simulink library "library_BCM"  (Simulink 8.2)
settings: Solver=ode45  StartTime=0.0  StopTime=10.0  RelTol=1e-3
undefined symbols (not defined in the file or in its folder): MPU_FOUR_CST, MPU_ONE_CST, MPU_THREE_CST, MPU_TWO_CST, MPU_ZERO_CST, NAMEOFTHEMODEL_SAMPLE_TIME_CST, slcm, TYP_MPU_REQUEST, TYP_MPU_REQUEST_2, TYP_MPU_STATUS, TYP_MPU_STATUS_2
libraries: Renault_Library x50, simulink x8, library_BCM x7
(part 2 of 3)

== system library_BCM/Modeling/PRESOAK_CHARGE_5CAL_7DAY ==
  IN_Prog_time : Inport
  CURENT_TIME : Inport  Port=2
  ONE_WEEK_IN_MINUTES : Inport  Port=3
  RelationalOperator : RelationalOperator  Operator=>  OutDataTypeStr=boolean  InputSameDT=on
  Subtract : Sum  Inputs=+-  OutDataTypeStr=Inherit: Inherit via back propagation  RndMeth=Zero  InputSameDT=on
  Sum : Sum  Inputs=++-  OutDataTypeStr=Inherit: Inherit via back propagation  RndMeth=Zero  InputSameDT=on
  Switch1 : Switch  Criteria=u2 ~= 0  RndMeth=Zero  InputSameDT=on
      settings: AttributesFormatString=Criteria=%<Criteria>
  Out_WUP : Outport
  wires:
  ONE_WEEK_IN_MINUTES/1 -> Sum/2
  Switch1/1 -> Out_WUP/1
  Sum/1 -> Switch1/3
  [CURENT_TIME] -> Sum/3
  [Prog_time] -> Sum/1
  [CURENT_TIME] -> Subtract/2
  [Prog_time] -> Subtract/1
  Subtract/1 -> Switch1/1
  IN_Prog_time/1 -> [Prog_time]
  CURENT_TIME/1 -> [CURENT_TIME]
  [CURENT_TIME] -> RelationalOperator/2
  RelationalOperator/1 -> Switch1/2
  [Prog_time] -> RelationalOperator/1

== system library_BCM/Modeling/RSA_Dynamic2DLookupTable_V01_00 ==
  x : Inport
  y : Inport  Port=2
  x_breakpoints : Inport  Port=3
  y_breakpoints : Inport  Port=4
  table : Inport  Port=5
  InterpolationUsingPrelookup : Interpolation_n-D  TableSource=Input port  ExtrapMethod=Clip  RndMeth=Zero
      settings: InputPortMap=u0,u1,u2,u3,p2
  Prelookup : PreLookup  BreakpointsDataSource=Input port  BreakpointsData=[1:4]  RndMeth=Zero
      settings: InputPortMap=u0,p1
  Prelookup1 : PreLookup  BreakpointsDataSource=Input port  BreakpointsData=[1:4]  RndMeth=Zero
      settings: InputPortMap=u0,p1
  Out : Outport
  wires:
  x/1 -> Prelookup/1
  InterpolationUsingPrelookup/1 -> Out/1
  table/1 -> InterpolationUsingPrelookup/5
  y/1 -> Prelookup1/1
  x_breakpoints/1 -> Prelookup/2
  y_breakpoints/1 -> Prelookup1/2
  Prelookup/2 -> InterpolationUsingPrelookup/2
  Prelookup/1 -> InterpolationUsingPrelookup/1
  Prelookup1/2 -> InterpolationUsingPrelookup/4
  Prelookup1/1 -> InterpolationUsingPrelookup/3

== system library_BCM/Modeling/TIME_OUT ==
  In : Inport  OutDataTypeStr=boolean
  dly : Inport  Port=2
  Constant1 : Constant  OutDataTypeStr=Inherit: Inherit via back propagation  SampleTime=-1
  Constant4 : Constant  Value=Ps  SampleTime=-1
  Constant9 : Constant  Value=INIVAL  SampleTime=-1
  DataTypeConversion : DataTypeConversion  OutDataTypeStr=uint32  RndMeth=Zero
  LogicalOperator1 : Logic  Operator=NOT  OutDataTypeStr=boolean
  MinMax : MinMax  Tag=AM,Std,Inputs,1;CMP,Function,Inputs;  Inputs=2  OutDataTypeStr=Inherit: Inherit via back propagation  RndMeth=Zero  SaturateOnIntegerOverflow=on  InputSameDT=on
  MinMax1 : MinMax  Tag=AM,Std,Inputs,1;CMP,Function,Inputs;  Function=max  Inputs=2  OutDataTypeStr=Inherit: Inherit via back propagation  RndMeth=Zero  SaturateOnIntegerOverflow=on  InputSameDT=on
  RSA_DetectDecrease : Renault_Library/Complex blocks/Logic & Bit Operations/RSA_DetectDecrease  Tag=[LIB]  vinit=false
      settings: AttributesFormatString=%<MaskType> : Ver : 01.02\nInitial condition: %<vinit>
  RelationalOperator1 : RelationalOperator  Tag=AM,Std,2,1;CMP,Operator;  Operator===  OutDataTypeStr=boolean  InputSameDT=on
  Sum1 : Sum  OutDataTypeStr=Inherit: Inherit via back propagation  RndMeth=Zero  SaturateOnIntegerOverflow=on  InputSameDT=on
  Sum2 : Sum  Inputs=+-  OutDataTypeStr=Inherit: Inherit via back propagation  RndMeth=Zero  SaturateOnIntegerOverflow=on  InputSameDT=on
  Sum3 : Sum  Inputs=+-  OutDataTypeStr=Inherit: Inherit via back propagation  RndMeth=Zero  SaturateOnIntegerOverflow=on  InputSameDT=on
  Switch1 : Switch  Criteria=u2 ~= 0  RndMeth=Zero  SaturateOnIntegerOverflow=on  InputSameDT=on
      settings: AttributesFormatString=Criteria=%<Criteria>
  UnitDelay : UnitDelay  InitialCondition=InitialConditions  SampleTime=-1
      settings: AttributesFormatString=IC = %<X0>
  UnitDelay1 : UnitDelay  InitialCondition=UDVAL  SampleTime=-1
      settings: AttributesFormatString=IC = %<X0>
  Out : Outport
  wires:
  Constant1/1 -> Sum3/2
  Sum3/1 -> DataTypeConversion/1
  dly/1 -> Sum3/1
  UnitDelay/1 -> Out/1
  LogicalOperator1/1 -> RSA_DetectDecrease/1
  RelationalOperator1/1 -> LogicalOperator1/1
  MinMax1/1 -> RelationalOperator1/1
  [Nsx_Zero] -> RelationalOperator1/2, MinMax1/2
  Sum2/1 -> MinMax/2
  MinMax/1 -> MinMax1/1
  In/1 -> Switch1/2
  Constant9/1 -> [Nsx_Zero], Switch1/1
  Sum1/1 -> Switch1/3
  UnitDelay1/1 -> Sum1/2
  Switch1/1 -> Sum2/2, UnitDelay1/1
  Constant4/1 -> Sum1/1
  DataTypeConversion/1 -> MinMax/1, Sum2/1
  RSA_DetectDecrease/1 -> UnitDelay/1

== system library_BCM/Modeling/Timer_Conversion ==
  TIMER_TO_ADAPT : Inport
      settings: AttributesFormatString=Type : %<OutDataTypeStr>
  Constant1 : Constant  Value=NAMEOFTHEMODEL_SAMPLE_TIME_CST  OutDataTypeStr=uint8  SampleTime=-1
  Constant2 : Constant  Value=NAMEOFTHEMODEL_SAMPLE_TIME_CST  OutDataTypeStr=Inherit: Inherit via back propagation  SampleTime=-1
  Constant3 : Constant  Value=ZERO_CST  OutDataTypeStr=Inherit: Inherit via back propagation  SampleTime=-1
  Divide : Product  Inputs=*/  SaturateOnIntegerOverflow=on  RndMeth=Zero  InputSameDT=on
      settings: AttributesFormatString=Saturation:%<SaturateOnIntegerOverflow>
  RelationalOperator1 : RelationalOperator  Operator===  OutDataTypeStr=boolean  InputSameDT=on
  Switch : Switch  Criteria=u2 ~= 0  RndMeth=Zero  InputSameDT=on
      settings: AttributesFormatString=Criteria=%<Criteria>
  TIMER_ADAPTED : Outport
      settings: AttributesFormatString=Type : %<OutDataTypeStr>\nInit :%<InitialOutput>
  wires:
  Divide/1 -> Switch/3
  [TIMER_TO_ADAPT] -> Divide/1
  [TIMER_TO_ADAPT] -> Switch/1
  TIMER_TO_ADAPT/1 -> [TIMER_TO_ADAPT]
  Switch/1 -> TIMER_ADAPTED/1
  RelationalOperator1/1 -> Switch/2
  Constant3/1 -> RelationalOperator1/2
  Constant1/1 -> RelationalOperator1/1
  Constant2/1 -> Divide/2

== system library_BCM/Validation/EEPROM ==
  EEPROM_S : Inport
  EEPROM_S_OUT : Inport  Port=2
  ECU_RESET : Inport  Port=3
  Data Store Memory : DataStoreMemory  DataStoreName=EEPROM_S  ReadBeforeWriteMsg=warning  WriteAfterWriteMsg=warning  WriteAfterReadMsg=warning
  DataStoreRead : Subsystem
      mask Display: fprintf('DataStoreRead')
  DataStoreWrite : Subsystem
      mask Display: fprintf('DataStoreWrite')
  EEPROM_S_IN : Outport
  wires:
  DataStoreRead/1(EEPROM_S_N) -> EEPROM_S_IN/1
  EEPROM_S_OUT/1 -> DataStoreWrite/2(EEPROM_S_OUT)
  EEPROM_S/1 -> DataStoreWrite/1(EEPROM_S)
  ECU_RESET/1 -> DataStoreWrite/3(ECU_RESET)

== system library_BCM/Validation/EEPROM_OLD ==
  READ : Inport
  WRITE : Inport  Port=2
  Chart : Stateflow chart  TreatAsAtomicUnit=on
  MultiportSwitch : MultiPortSwitch  Inputs=2
  S_IN : Outport
  wires:
  Chart/1(x) -> MultiportSwitch/1
  READ/1 -> MultiportSwitch/2, Chart/1(READ)
  WRITE/1 -> MultiportSwitch/3, Chart/2(WRITE)
  MultiportSwitch/1 -> S_IN/1

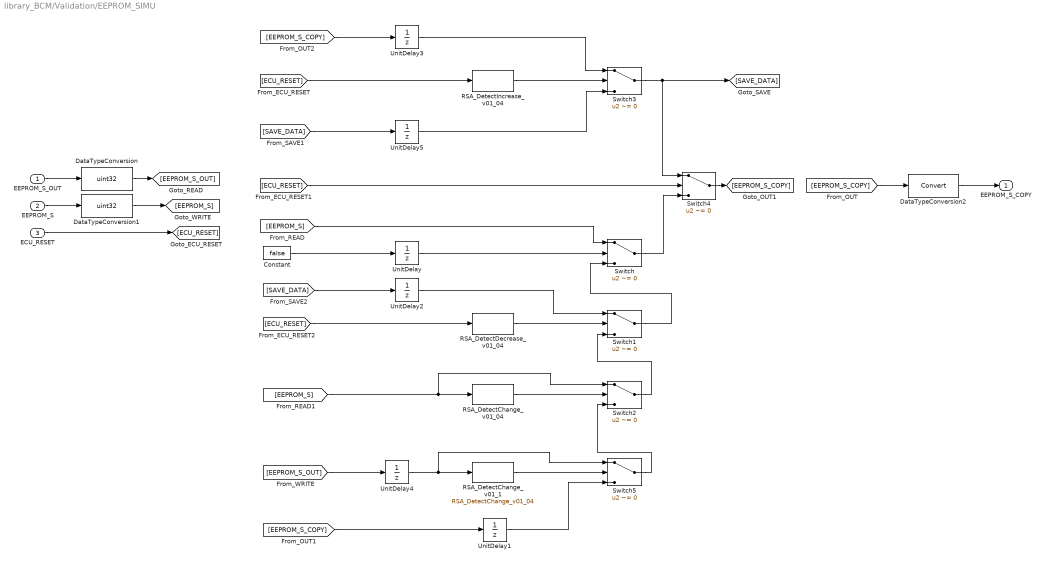
== system library_BCM/Validation/EEPROM_SIMU ==
  EEPROM_S_OUT : Inport
  EEPROM_S : Inport  Port=2
  ECU_RESET : Inport  Port=3
  Constant : Constant  Value=false  OutDataTypeStr=boolean  SampleTime=-1
  DataTypeConversion : DataTypeConversion  OutDataTypeStr=uint32  RndMeth=Zero
      settings: AttributesFormatString=Saturation:%<SaturateOnIntegerOverflow>
  DataTypeConversion1 : DataTypeConversion  OutDataTypeStr=uint32  RndMeth=Zero
      settings: AttributesFormatString=Saturation:%<SaturateOnIntegerOverflow>
  DataTypeConversion2 : DataTypeConversion  RndMeth=Zero
      settings: AttributesFormatString=Saturation:%<SaturateOnIntegerOverflow>
  RSA_DetectChange_v01_04 : Renault_Library/Complex blocks/Logic & Bit Operations/RSA_DetectChange_v01_04  Tag=[LIB]  chkini=off  vinit=0
      settings: AttributesFormatString=%<MaskType> : Ver : 01.04\nCompare the Input with Initial Value = %<chkini>\nInitial Value : = %<vinit>
  RSA_DetectChange_v01_1 : Renault_Library/Complex blocks/Logic & Bit Operations/RSA_DetectChange_v01_04  Tag=[LIB]  chkini=off  vinit=0
      settings: AttributesFormatString=%<MaskType> : Ver : 01.04\nCompare the Input with Initial Value = %<chkini>\nInitial Value : = %<vinit>
  RSA_DetectDecrease_v01_04 : Renault_Library/Complex blocks/Logic & Bit Operations/RSA_DetectDecrease_v01_04  Tag=[LIB]  chkini=on  vinit=0
      settings: AttributesFormatString=%<MaskType> : Ver : 01.04\nCompare the Input with Initial Value = %<chkini>\nInitial Value : = %<vinit>
  RSA_DetectIncrease_v01_04 : Renault_Library/Complex blocks/Logic & Bit Operations/RSA_DetectIncrease_v01_04  Tag=[LIB]  chkini=off  vinit=false
      settings: AttributesFormatString=%<MaskType> : Ver : 01.04\nCompare the Input with Initial Value = %<chkini>\nInitial Value : = %<vinit>
  Switch{,1..5} (6 alike) : Switch  Criteria=u2 ~= 0  RndMeth=Zero  InputSameDT=on
      settings: AttributesFormatString=Criteria=%<Criteria>
  UnitDelay : UnitDelay  InitialCondition=true  SampleTime=-1
      settings: AttributesFormatString=IC = %<X0>
  UnitDelay{1..5} (5 alike) : UnitDelay  SampleTime=-1
      settings: AttributesFormatString=IC = %<X0>
  EEPROM_S_COPY : Outport
  wires:
  DataTypeConversion2/1 -> EEPROM_S_COPY/1
  DataTypeConversion1/1 -> [EEPROM_S]
  DataTypeConversion/1 -> [EEPROM_S_OUT]
  [ECU_RESET] -> Switch4/2
  Switch/1 -> Switch4/3
  UnitDelay5/1 -> Switch3/3
  [SAVE_DATA] -> UnitDelay5/1
  UnitDelay3/1 -> Switch3/1
  RSA_DetectIncrease_v01_04/1 -> Switch3/2
  Switch3/1 -> [SAVE_DATA], Switch4/1
  Switch4/1 -> [EEPROM_S_COPY]
  [EEPROM_S_COPY] -> UnitDelay3/1
  [ECU_RESET] -> RSA_DetectIncrease_v01_04/1
  ECU_RESET/1 -> [ECU_RESET]
  EEPROM_S/1 -> DataTypeConversion1/1
  EEPROM_S_OUT/1 -> DataTypeConversion/1
  [EEPROM_S_COPY] -> DataTypeConversion2/1
  Constant/1 -> UnitDelay/1
  UnitDelay/1 -> Switch/2
  [EEPROM_S] -> Switch/1
  RSA_DetectChange_v01_04/1 -> Switch2/2
  [EEPROM_S] -> Switch2/1, RSA_DetectChange_v01_04/1
  [ECU_RESET] -> RSA_DetectDecrease_v01_04/1
  RSA_DetectDecrease_v01_04/1 -> Switch1/2
  [SAVE_DATA] -> UnitDelay2/1
  UnitDelay2/1 -> Switch1/1
  Switch1/1 -> Switch/3
  Switch2/1 -> Switch1/3
  [EEPROM_S_OUT] -> UnitDelay4/1
  RSA_DetectChange_v01_1/1 -> Switch5/2
  Switch5/1 -> Switch2/3
  [EEPROM_S_COPY] -> UnitDelay1/1
  UnitDelay1/1 -> Switch5/3
  UnitDelay4/1 -> Switch5/1, RSA_DetectChange_v01_1/1

== system library_BCM/Fault Manager/DTC/DETECT_DTC_IN_E2P_FOR_RESET ==
  FailureConfirmed : Inport  OutDataTypeStr=boolean
      settings: AttributesFormatString=Type : %<OutDataTypeStr>
  DTC_LIST_OUT_EXT_DATA_S : Inport  Port=2  OutDataTypeStr=uint32
      settings: AttributesFormatString=Type : %<OutDataTypeStr>
  NUMBER_DTC_RECORD_IN_E2P_CST : Inport  Port=3  OutDataTypeStr=uint32
      settings: AttributesFormatString=Type : %<OutDataTypeStr>
  DTC_LIST_OUT_IDENTITY_DTC_S : Inport  Port=4  OutDataTypeStr=uint32
      settings: AttributesFormatString=Type : %<OutDataTypeStr>
  DTC_ID : Inport  Port=5  OutDataTypeStr=uint32
      settings: AttributesFormatString=Type : %<OutDataTypeStr>
  Enable : EnablePort
      settings: AttributesFormatString=State : %<StatesWhenEnabling>
  ForIteratorSubsystem : Subsystem  TreatAsAtomicUnit=on
  TO_ADD_1_CALCUL_IN_LOOP : Subsystem
  ExtendedData_reset : Outport  OutDataTypeStr=uint32  InitialOutput=0
      settings: CopyFcn=if exist('tl_check_ports','file'), tl_check_ports(gcbh); end  NameChangeFcn=if exist('tl_check_ports','file'), tl_check_ports(gcbh); end
  wires:
  FailureConfirmed/1 -> ForIteratorSubsystem/5(FailureConfirmed)
  DTC_ID/1 -> ForIteratorSubsystem/4(DTC_ID)
  DTC_LIST_OUT_IDENTITY_DTC_S/1 -> ForIteratorSubsystem/3(DTC_LIST_OUT_IDENTITY_DTC_S)
  DTC_LIST_OUT_EXT_DATA_S/1 -> ForIteratorSubsystem/2(DTC_LIST_OUT_EXT_DATA_S)
  ForIteratorSubsystem/1(ExtendedData) -> ExtendedData_reset/1
  TO_ADD_1_CALCUL_IN_LOOP/1(NB_DTC_RECORD_IN_E2P_CST_EXT) -> [NB_DTC_RECORD_IN_E2P_CST_EXT]
  NUMBER_DTC_RECORD_IN_E2P_CST/1 -> TO_ADD_1_CALCUL_IN_LOOP/1(NUMBER_DTC_RECORD_IN_E2P_CST)
  [NB_DTC_RECORD_IN_E2P_CST_EXT] -> ForIteratorSubsystem/1(NUMBER_DTC_RECORD_IN_E2P_CST)

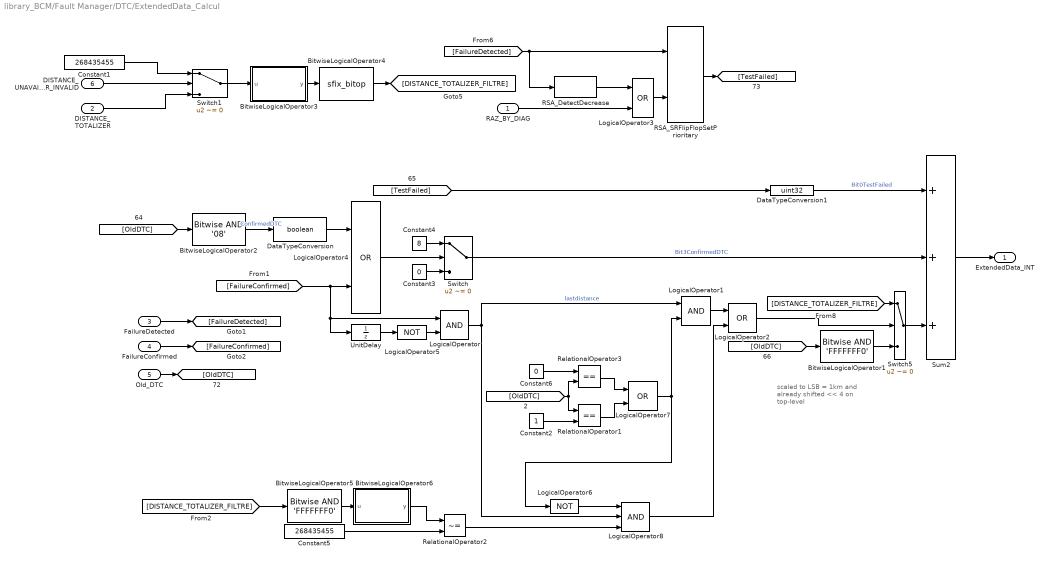
== system library_BCM/Fault Manager/DTC/ExtendedData_Calcul ==
  note: scaled to LSB = 1km
      | and already shifted << 4
      | on top-level
  RAZ_BY_DIAG : Inport  OutDataTypeStr=boolean
  DISTANCE_TOTALIZER : Inport  Port=2  OutDataTypeStr=uint32
      settings: CopyFcn=if exist('tl_check_ports','file'), tl_check_ports(gcbh); end  NameChangeFcn=if exist('tl_check_ports','file'), tl_check_ports(gcbh); end
  FailureDetected : Inport  Port=3  OutDataTypeStr=boolean
  FailureConfirmed : Inport  Port=4  OutDataTypeStr=boolean
  Old_DTC : Inport  Port=5  OutDataTypeStr=uint32
  DISTANCE_UNAVAILABLE_OR_INVALID : Inport  Port=6  OutDataTypeStr=boolean
  BitwiseLogicalOperator1 : simulink/Logic and Bit Operations/Bitwise Operator  Tag=struct('revisionNumber',2,'output',struct('type','UInt32'),'operator','AND','operand2','''FFFFFF00''','numInput',1)  logicop=AND  UseBitMask=on  BitMask='FFFFFFF0'  BitMaskRealWorld=Stored Integer
  BitwiseLogicalOperator2 : simulink/Logic and Bit Operations/Bitwise Operator  Tag=struct('revisionNumber',2,'output',struct('type','UInt8'),'operator','AND','operand2','''08''','numInput',1)  logicop=AND  UseBitMask=on  BitMask='08'  BitMaskRealWorld=Stored Integer
  BitwiseLogicalOperator3 : Subsystem  Tag=struct('revisionNumber',2,'output',struct('type','UInt32'),'operator','SHIFT_LEFT','operand2','8','numInput',1)  mask(Shift Arithmetic){nBitShiftRight=-4, nBinPtShiftRight=0}
      mask prompts: nBitShiftRight "Number of bits to shift right (use negative value to shift left):"; nBinPtShiftRight "Number of places by which binary point shifts right (use negative value to shift left):"
      mask help:
      | This block can arithmetically shift the bits and/or the binary point of a signal.
      | The effect of these actions can be interpreted as a combination of a multiplication by a power of two and a change in scaling.  The power of two multiplication term is
      |   2^( NumBinaryPointShiftsRight - NumBitShiftsRight )
      | Negative values for shifts right are actually positive shift lefts.
      | If the input is a floating point type, the power of two multiplication is carried out, but no change in scaling is applied.
      mask init:
      | netExponent = nBinPtShiftRight - nBitShiftRight;
      | netExponent(find(netExponent>127)) = 127;
      | netExponent(find(netExponent<-127)) = -127;
      | nBitShiftRight(find(nBitShiftRight>127)) = 127;
      | nBitShiftRight(find(nBitShiftRight<-127)) = -127;
      | dstr = ['Vy = Vu'];
      | if netExponent ~= 0
      |   dstr = [dstr,' * 2^',num2str(netExponent)];
      | end
      | dstr = [dstr,'\nQy = Qu'];
      | if nBitShiftRight > 0
      |   dstr = [dstr,' >> ',num2str(nBitShiftRight)];
      | elseif nBitShiftRight < 0
      |  dstr = [dstr,' << ',num2str(-nBitShiftRight)];
      | end
      | dstr = [dstr,'\nEy = Eu'];
      | if nBinPtShiftRight > 0
      |   dstr = [dstr,' + ',num2str(nBinPtShiftRight)];
      | elseif nBinPtShiftRight < 0
      |   dstr = [dstr,' - ',num2str(-nBinPtShiftRight)];
      | end
      | for i = 1:length(netExponent)
      |     netExponent(i) = 2^netExponent(i);
      | end
      mask Display: fprintf(dstr)
  BitwiseLogicalOperator4 : S-Function  Tag=struct('revisionNumber',2,'output',struct('type','UInt32'),'operator','AND','operand2','''FFFFFF00''','numInput',1)  FunctionName=sfix_bitop  Parameters=UseBitMask,NumInputPorts,BitMask,BitMaskRealWorld,logicop  EnableBusSupport=off  mask(Bitwise Operator){logicop=AND, UseBitMask=on, NumInputPorts=1, BitMask='FFFFFFF0', BitMaskRealWorld=Stored Integer}
      mask prompts: logicop "Operator:"; UseBitMask "Use bit mask ..."; NumInputPorts "Number of input ports:"; BitMask "Bit Mask"; BitMaskRealWorld "Treat mask as:"
      mask help: Perform the specified bitwise operation on the inputs. The output data type should represent zero exactly.
      mask init:
      | if UseBitMask
      |   [m,n] = size(BitMask);
      |   if ischar(BitMask)
      |     len = m;
      |     n = 1;
      |   else
      |     len = m * n;
      |   end
      |   internalBitMask = zeros(m,n);
      |   if isnumeric(BitMask)
      |     for i=1:len,
      |       internalBitMask(i) = BitMask(i);
      |     end
      |   elseif ischar(BitMask)
      |     for i=1:m,
      |       internalBitMask(i) = hex2dec(BitMask(i,:));
      |     end
      |   elseif iscell(BitMask)
      |     for i=1:len,
      |       if isnumeric( BitMask{i} )
      |         internalBitMask(i) = BitMask{i};
      |       elseif ischar( BitMask{i} )
      |         internalBitMask(i) = hex2dec(BitMask{i});
      |       else
      |         errordlg(['Data type is not supported at cell item ', num2str(i) ]);
      |       end
      |     end
      |   end
      |   BitMask = internalBitMask;
      |   if len == 1
      |      if BitMaskRealWorld == 1 || BitMask(1) < 0
      |        str=num2str(BitMask(1));
      |      else
      |        str=['0x',dec2hex(floor(BitMask(1)))];
      |      end
      |   else
      |      str='Masks';
      |   end
      | else
      |   BitMask = 0;
      |   str='';
      | end
      mask TypeOptions logicop: AND | OR | NAND | NOR | XOR | NOT
      mask Callback logicop: fixptdialog(gcbh)
      mask Callback UseBitMask: fixptdialog(gcbh)
      mask TypeOptions BitMaskRealWorld: Real World Value | Stored Integer
      mask Display: fprintf(['Bitwise\n',logicop,'\n',str])
  BitwiseLogicalOperator5 : simulink/Logic and Bit Operations/Bitwise Operator  Tag=struct('revisionNumber',2,'output',struct('type','UInt32'),'operator','AND','operand2','''FFFFFF00''','numInput',1)  logicop=AND  UseBitMask=on  BitMask='FFFFFFF0'  BitMaskRealWorld=Stored Integer
  BitwiseLogicalOperator6 : Subsystem  Tag=struct('revisionNumber',2,'output',struct('type','UInt32'),'operator','SHIFT_LEFT','operand2','8','numInput',1)  mask(Shift Arithmetic){nBitShiftRight=4, nBinPtShiftRight=0}
      mask prompts: nBitShiftRight "Number of bits to shift right (use negative value to shift left):"; nBinPtShiftRight "Number of places by which binary point shifts right (use negative value to shift left):"
      mask help:
      | This block can arithmetically shift the bits and/or the binary point of a signal.
      | The effect of these actions can be interpreted as a combination of a multiplication by a power of two and a change in scaling.  The power of two multiplication term is
      |   2^( NumBinaryPointShiftsRight - NumBitShiftsRight )
      | Negative values for shifts right are actually positive shift lefts.
      | If the input is a floating point type, the power of two multiplication is carried out, but no change in scaling is applied.
      mask init: same as library_BCM/Fault Manager/DTC/ExtendedData_Calcul/BitwiseLogicalOperator3
      mask Display: fprintf(dstr)
  Constant1 : Constant  Value=268435455  OutDataTypeStr=uint32  SampleTime=-1
  Constant2 : Constant  Tag=struct('comment',struct('text','','placement',1),'output',struct('variable','','description','','name','$S_$B','width',1,'address','','max',NaN,'min',NaN,'class','default','type','UInt8','scaling','','lsb',1,'offset',0,'arb',0,'freeze',1,'unit','','keepdatatype',1,'value','0','tolerance',1,'castoutput',0,'show',0),'dt','0.02','scalingvalid',0,'date',733414.67771248845)  OutDataTypeStr=uint32  SampleTime=-1
  Constant3 : Constant  Tag=struct('comment',struct('text','','placement',1),'output',struct('variable','','description','','name','$S_$B','width',1,'address','','max',NaN,'min',NaN,'class','default','type','UInt8','scaling','','lsb',1,'offset',0,'arb',0,'freeze',1,'unit','','keepdatatype',1,'value','0','tolerance',1,'castoutput',0,'show',0),'dt','0.02','scalingvalid',0,'date',733414.67771248845)  Value=0  OutDataTypeStr=uint32  SampleTime=-1
  Constant4 : Constant  Tag=struct('comment',struct('text','','placement',1),'output',struct('variable','','description','','name','$S_$B','width',1,'address','','max',NaN,'min',NaN,'class','default','type','UInt8','scaling','','lsb',1,'offset',0,'arb',0,'freeze',1,'unit','','keepdatatype',1,'value','0','tolerance',1,'castoutput',0,'show',0),'dt','0.02','scalingvalid',0,'date',733414.67771248845)  Value=8  OutDataTypeStr=uint32  SampleTime=-1
  Constant5 : Constant  Value=268435455  OutDataTypeStr=uint32  SampleTime=-1
  Constant6 : Constant  Tag=struct('comment',struct('text','','placement',1),'output',struct('variable','','description','','name','$S_$B','width',1,'address','','max',NaN,'min',NaN,'class','default','type','UInt8','scaling','','lsb',1,'offset',0,'arb',0,'freeze',1,'unit','','keepdatatype',1,'value','0','tolerance',1,'castoutput',0,'show',0),'dt','0.02','scalingvalid',0,'date',733414.67771248845)  Value=0  OutDataTypeStr=uint32  SampleTime=-1
  DataTypeConversion : DataTypeConversion  OutDataTypeStr=boolean  RndMeth=Zero
      settings: AttributesFormatString=Saturation:%<SaturateOnIntegerOverflow>
  DataTypeConversion1 : DataTypeConversion  OutDataTypeStr=uint32  RndMeth=Zero
  LogicalOperator : Logic  Tag=struct('inputs','2','comment',struct('text','','placement',1),'logdata',struct('maxnumvals',inf,'plotchannels',[],'loggingmode',3,'channels',1),'operator','AND','output',struct('variable','','description','','name','$S_$B','address','','class','default','type','Bool','unit',''),'scalingvalid',0,'date',730486)  OutDataTypeStr=boolean
  LogicalOperator1 : Logic  Tag=struct('inputs','2','comment',struct('text','','placement',1),'logdata',struct('maxnumvals',inf,'plotchannels',[],'loggingmode',3,'channels',1),'operator','AND','output',struct('variable','','description','','name','$S_$B','address','','class','default','type','Bool','unit',''),'scalingvalid',0,'date',730486)  OutDataTypeStr=boolean
  LogicalOperator2 : Logic  Tag=struct('inputs','2','comment',struct('text','','placement',1),'logdata',struct('maxnumvals',inf,'plotchannels',[],'loggingmode',3,'channels',1),'operator','AND','output',struct('variable','','description','','name','$S_$B','address','','class','default','type','Bool','unit',''),'scalingvalid',0,'date',730486)  Operator=OR  OutDataTypeStr=boolean
  LogicalOperator3 : Logic  Operator=OR  OutDataTypeStr=boolean
  LogicalOperator4 : Logic  Operator=OR  OutDataTypeStr=boolean
  LogicalOperator5 : Logic  Operator=NOT  OutDataTypeStr=boolean
  LogicalOperator6 : Logic  Operator=NOT  OutDataTypeStr=boolean
  LogicalOperator7 : Logic  Tag=struct('inputs','2','comment',struct('text','','placement',1),'logdata',struct('maxnumvals',inf,'plotchannels',[],'loggingmode',3,'channels',1),'operator','AND','output',struct('variable','','description','','name','$S_$B','address','','class','default','type','Bool','unit',''),'scalingvalid',0,'date',730486)  Operator=OR  OutDataTypeStr=boolean
  LogicalOperator8 : Logic  Tag=struct('inputs','2','comment',struct('text','','placement',1),'logdata',struct('maxnumvals',inf,'plotchannels',[],'loggingmode',3,'channels',1),'operator','AND','output',struct('variable','','description','','name','$S_$B','address','','class','default','type','Bool','unit',''),'scalingvalid',0,'date',730486)  Inputs=3  OutDataTypeStr=boolean
  RSA_DetectDecrease : Renault_Library/Complex blocks/Logic & Bit Operations/RSA_DetectDecrease  Tag=[LIB]  vinit=0
      settings: AttributesFormatString=%<MaskType> : Ver : 01.02\nInitial condition: %<vinit>
  RSA_SRFlipFlopSetPrioritary : Renault_Library/Complex blocks/Flip-Flop/RSA_SRFlipFlopSetPrioritary  Tag=[LIB]  init=false
      settings: AttributesFormatString=%<MaskType> : Ver : 01.02\n<init=%<init>>
  RelationalOperator1 : RelationalOperator  Operator===  OutDataTypeStr=boolean  InputSameDT=on
  RelationalOperator2 : RelationalOperator  Operator=~=  OutDataTypeStr=boolean  InputSameDT=on
  RelationalOperator3 : RelationalOperator  Operator===  OutDataTypeStr=boolean  InputSameDT=on
  Sum2 : Sum  Tag=struct('comment',struct('text','','placement',1),'logdata',struct('maxnumvals',inf,'plotchannels',[],'loggingmode',3,'channels',1),'output',struct('variable','','description','','name','$S_$B','width',1,'address','','max',NaN,'min',NaN,'class','default','type','UInt8','scaling','','lsb',1,'offset',0,'arb',0,'freeze',1,'unit','','autoscalingmode',1,'lowerheadroom',1,'upperheadroom',1,'headroomunit','bit','keepdatatype',1,'checkmin',0,'checkmax',0,'castoutput',0,'show',0),'inputs','+++++','scalingvalid',0,'date',732947.44426018524)  Inputs=+++  RndMeth=Zero
  Switch : Switch  Tag=struct('comment',struct('text','','placement',1),'logdata',struct('maxnumvals',inf,'plotchannels',[],'loggingmode',3,'channels',1),'output',struct('variable','','description','','name','$S_$B','width',1,'address','','max',255,'min',0,'class','default','type','UInt8','scaling','','lsb',1,'offset',0,'arb',0,'freeze',1,'unit','','autoscalingmode',1,'lowerheadroom',1,'upperheadroom',1,'headroomunit','bit','keepdatatype',1,'checkmin',0,'checkmax',0,'castoutput',0,'show',0),'inheritscaling',0,'threshold',struct('variable','','description','','name','$S_$B_threshold','width',1,'address','','max',NaN,'min',NaN,'class','default','type','Int16','scaling','','lsb',1,'offset',0,'arb',0,'freeze',1,'unit','','keepdatatype',1,'value','0','scalar',0,'criteria',3),'scalingvalid',0,'date',733414.64197635418)  Criteria=u2 ~= 0  OutDataTypeStr=uint32  RndMeth=Zero  SaturateOnIntegerOverflow=on  InputSameDT=on
      settings: AttributesFormatString=Criteria=%<Criteria>
  Switch1 : Switch  Criteria=u2 ~= 0  RndMeth=Zero  InputSameDT=on
      settings: AttributesFormatString=Criteria=%<Criteria>
  Switch5 : Switch  Tag=struct('comment',struct('text','','placement',1),'logdata',struct('maxnumvals',inf,'plotchannels',[],'loggingmode',3,'channels',1),'output',struct('variable','','description','','name','$S_$B','width',1,'address','','max',NaN,'min',NaN,'class','default','type','UInt32','scaling','','lsb',1,'offset',0,'arb',0,'freeze',1,'unit','','autoscalingmode',1,'lowerheadroom',1,'upperheadroom',1,'headroomunit','bit','keepdatatype',1,'checkmin',0,'checkmax',0,'castoutput',0,'show',0),'inheritscaling',0,'threshold',struct('variable','','description','','name','$S_$B_threshold','width',1,'address','','max',NaN,'min',NaN,'class','default','type','Int16','scaling','','lsb',1,'offset',0,'arb',0,'freeze',1,'unit','','keepdatatype',1,'value','0','scalar',0,'criteria',3),'scalingvalid',0,'date',733414.68391717598)  Criteria=u2 ~= 0  RndMeth=Zero  SaturateOnIntegerOverflow=on  InputSameDT=on
      settings: AttributesFormatString=Criteria=%<Criteria>
  UnitDelay : UnitDelay  Tag=struct('comment',struct('text','','placement',1),'logdata',struct('maxnumvals',inf,'plotchannels',[],'loggingmode',3,'channels',inf),'output',struct('variable','','description','','name','$S_$B','width',1,'address','','max',NaN,'min',NaN,'class','default','type','Int16','scaling','','lsb',1,'offset',0,'arb',0,'freeze',1,'unit','','autoscalingmode',1,'lowerheadroom',1,'upperheadroom',1,'headroomunit','bit','keepdatatype',1,'checkmin',0,'checkmax',0,'castoutput',0,'show',0),'inheritscaling',1,'state',struct('variable','','description','','name','X_$S_$B','width',1,'address','','max',NaN,'min',NaN,'class','default','type','Int16','scaling','','lsb',1,'offset',0,'arb',0,'freeze',1,'unit','','initial','0'),'dt','-1','scalingvalid',0,'date',733303.57871097222)  SampleTime=-1
      settings: AttributesFormatString=IC = %<X0>
  ExtendedData_INT : Outport  OutDataTypeStr=uint32  InitialOutput=0
      settings: CopyFcn=if exist('tl_check_ports','file'), tl_check_ports(gcbh); end  NameChangeFcn=if exist('tl_check_ports','file'), tl_check_ports(gcbh); end
  wires:
  DataTypeConversion/1 -> LogicalOperator4/1
  Old_DTC/1 -> [OldDTC]
  Sum2/1 -> ExtendedData_INT/1
  FailureConfirmed/1 -> [FailureConfirmed]
  FailureDetected/1 -> [FailureDetected]
  BitwiseLogicalOperator4/1 -> [DISTANCE_TOTALIZER_FILTRE]
  BitwiseLogicalOperator3/1(y) -> BitwiseLogicalOperator4/1
  [FailureDetected] -> RSA_SRFlipFlopSetPrioritary/1, RSA_DetectDecrease/1
  Switch5/1 -> Sum2/3
  RSA_SRFlipFlopSetPrioritary/1 -> [TestFailed]
  LogicalOperator3/1 -> RSA_SRFlipFlopSetPrioritary/2
  RAZ_BY_DIAG/1 -> LogicalOperator3/2
  RSA_DetectDecrease/1 -> LogicalOperator3/1
  [TestFailed] -> DataTypeConversion1/1
  [OldDTC] -> BitwiseLogicalOperator1/1
  Constant3/1 -> Switch/3
  Constant4/1 -> Switch/1
  UnitDelay/1 -> LogicalOperator5/1
  LogicalOperator5/1 -> LogicalOperator/2
  LogicalOperator/1 -> LogicalOperator8/2, LogicalOperator1/1  "lastdistance"
  Switch/1 -> Sum2/2  "Bit3ConfirmedDTC"
  LogicalOperator4/1 -> Switch/2
  [DISTANCE_TOTALIZER_FILTRE] -> Switch5/1
  BitwiseLogicalOperator2/1 -> DataTypeConversion/1  "ConfirmedDTC"
  [OldDTC] -> BitwiseLogicalOperator2/1
  DataTypeConversion1/1 -> Sum2/1  "Bit0TestFailed"
  BitwiseLogicalOperator1/1 -> Switch5/3
  [FailureConfirmed] -> LogicalOperator4/2, LogicalOperator/1, UnitDelay/1
  DISTANCE_UNAVAILABLE_OR_INVALID/1 -> Switch1/2
  Switch1/1 -> BitwiseLogicalOperator3/1(u)
  DISTANCE_TOTALIZER/1 -> Switch1/3
  Constant1/1 -> Switch1/1
  LogicalOperator7/1 -> LogicalOperator1/2, LogicalOperator6/1
  [DISTANCE_TOTALIZER_FILTRE] -> BitwiseLogicalOperator5/1
  BitwiseLogicalOperator5/1 -> BitwiseLogicalOperator6/1(u)
  BitwiseLogicalOperator6/1(y) -> RelationalOperator2/1
  Constant5/1 -> RelationalOperator2/2
  LogicalOperator1/1 -> LogicalOperator2/1
  LogicalOperator2/1 -> Switch5/2
  RelationalOperator2/1 -> LogicalOperator8/3
  LogicalOperator8/1 -> LogicalOperator2/2
  LogicalOperator6/1 -> LogicalOperator8/1
  [OldDTC] -> RelationalOperator3/2, RelationalOperator1/1
  Constant6/1 -> RelationalOperator3/1
  Constant2/1 -> RelationalOperator1/2
  RelationalOperator3/1 -> LogicalOperator7/1
  RelationalOperator1/1 -> LogicalOperator7/2

== system library_BCM/Fault Manager/DTC/RAZ_AND_RESET ==
  ExtendedData_INT : Inport  OutDataTypeStr=uint32
      settings: AttributesFormatString=Type : %<OutDataTypeStr>
  RAZ_BY_DIAG : Inport  Port=2  OutDataTypeStr=boolean
      settings: AttributesFormatString=Type : %<OutDataTypeStr>
  CF : Inport  Port=3  OutDataTypeStr=boolean
      settings: AttributesFormatString=Type : %<OutDataTypeStr>
  ExtendedData_reset : Inport  Port=4  OutDataTypeStr=uint32
      settings: AttributesFormatString=Type : %<OutDataTypeStr>
  Constant8 : Constant  Value=false  OutDataTypeStr=boolean  SampleTime=-1
  Constant9 : Constant  Tag=struct('comment',struct('text','','placement',1),'output',struct('variable','','description','','name','$S_$B','width',1,'address','','max',NaN,'min',NaN,'class','default','type','UInt8','scaling','','lsb',1,'offset',0,'arb',0,'freeze',1,'unit','','keepdatatype',1,'value','0','tolerance',1,'castoutput',0,'show',0),'dt','0.02','scalingvalid',0,'date',733414.67771248845)  Value=0  OutDataTypeStr=uint32  SampleTime=-1
  LogicalOperator : Logic  Operator=OR  OutDataTypeStr=boolean
  LogicalOperator7 : Logic  Operator=NOT  OutDataTypeStr=boolean
  Switch1 : Switch  Tag=struct('comment',struct('text','','placement',1),'logdata',struct('maxnumvals',inf,'plotchannels',[],'loggingmode',3,'channels',1),'output',struct('variable','','description','','name','$S_$B','width',1,'address','','max',NaN,'min',NaN,'class','default','type','UInt32','scaling','','lsb',1,'offset',0,'arb',0,'freeze',1,'unit','','autoscalingmode',1,'lowerheadroom',1,'upperheadroom',1,'headroomunit','bit','keepdatatype',1,'checkmin',0,'checkmax',0,'castoutput',0,'show',0),'inheritscaling',0,'threshold',struct('variable','','description','','name','$S_$B_threshold','width',1,'address','','max',NaN,'min',NaN,'class','default','type','Int16','scaling','','lsb',1,'offset',0,'arb',0,'freeze',1,'unit','','keepdatatype',1,'value','0','scalar',0,'criteria',3),'scalingvalid',0,'date',733414.68413057865)  Criteria=u2 ~= 0  RndMeth=Zero  SaturateOnIntegerOverflow=on  InputSameDT=on
      settings: AttributesFormatString=Criteria=%<Criteria>
  Switch4 : Switch  Tag=struct('comment',struct('text','','placement',1),'logdata',struct('maxnumvals',inf,'plotchannels',[],'loggingmode',3,'channels',1),'output',struct('variable','','description','','name','$S_$B','width',1,'address','','max',NaN,'min',NaN,'class','default','type','UInt32','scaling','','lsb',1,'offset',0,'arb',0,'freeze',1,'unit','','autoscalingmode',1,'lowerheadroom',1,'upperheadroom',1,'headroomunit','bit','keepdatatype',1,'checkmin',0,'checkmax',0,'castoutput',0,'show',0),'inheritscaling',0,'threshold',struct('variable','','description','','name','$S_$B_threshold','width',1,'address','','max',NaN,'min',NaN,'class','default','type','Int16','scaling','','lsb',1,'offset',0,'arb',0,'freeze',1,'unit','','keepdatatype',1,'value','0','scalar',0,'criteria',3),'scalingvalid',0,'date',733414.68413057865)  Criteria=u2 ~= 0  RndMeth=Zero  SaturateOnIntegerOverflow=on  InputSameDT=on
      settings: AttributesFormatString=Criteria=%<Criteria>
  UnitDelay2 : UnitDelay  InitialCondition=1  SampleTime=-1
      settings: AttributesFormatString=IC = %<X0>
  ExtendedData : Outport
      settings: AttributesFormatString=Type : %<OutDataTypeStr>
  wires:
  ExtendedData_INT/1 -> Switch1/3
  ExtendedData_reset/1 -> Switch1/1
  UnitDelay2/1 -> Switch1/2
  Constant8/1 -> UnitDelay2/1
  Switch1/1 -> Switch4/3
  LogicalOperator/1 -> Switch4/2
  Switch4/1 -> ExtendedData/1
  Constant9/1 -> Switch4/1
  RAZ_BY_DIAG/1 -> LogicalOperator/1
  CF/1 -> LogicalOperator7/1
  LogicalOperator7/1 -> LogicalOperator/2

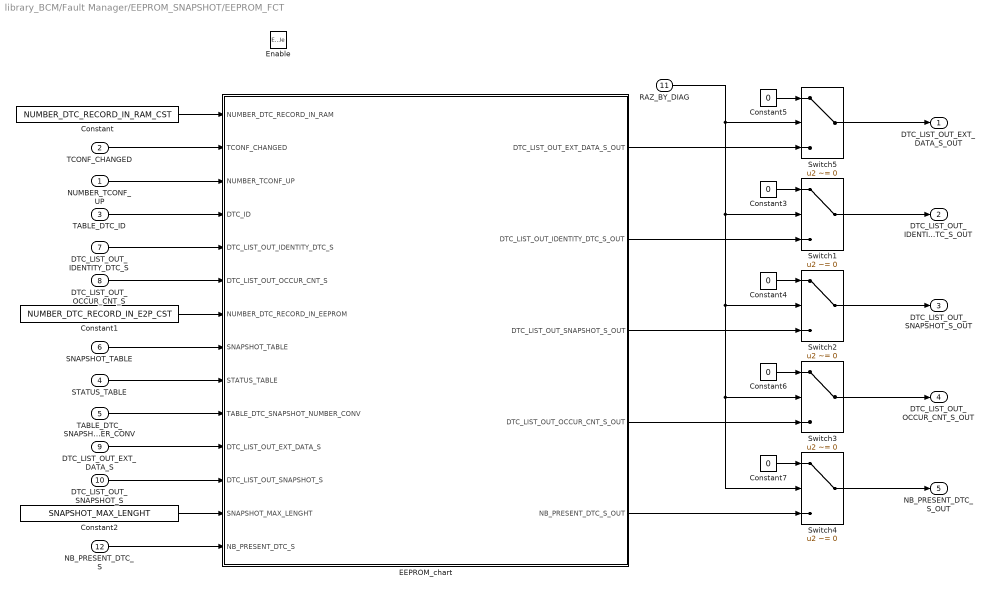
== system library_BCM/Fault Manager/EEPROM_SNAPSHOT/EEPROM_FCT ==
  NUMBER_TCONF_UP : Inport
  TCONF_CHANGED : Inport  Port=2
  TABLE_DTC_ID : Inport  Port=3  OutDataTypeStr=uint32
      settings: AttributesFormatString=Type : %<OutDataTypeStr>
  STATUS_TABLE : Inport  Port=4  OutDataTypeStr=uint32  PortDimensions=NUMBER_DTC_RECORD_IN_RAM_CST
      settings: AttributesFormatString=Type : %<OutDataTypeStr>
  TABLE_DTC_SNAPSHOT_NUMBER_CONV : Inport  Port=5  OutDataTypeStr=uint8  PortDimensions=NUMBER_DTC_RECORD_IN_RAM_CST
      settings: AttributesFormatString=Type : %<OutDataTypeStr>
  SNAPSHOT_TABLE : Inport  Port=6  OutDataTypeStr=uint8  PortDimensions=[SNAPSHOT_MAX_LENGHT SNAPSHOT_NUMBER_CST]
      settings: AttributesFormatString=Type : %<OutDataTypeStr>
  DTC_LIST_OUT_IDENTITY_DTC_S : Inport  Port=7
  DTC_LIST_OUT_OCCUR_CNT_S : Inport  Port=8
  DTC_LIST_OUT_EXT_DATA_S : Inport  Port=9
  DTC_LIST_OUT_SNAPSHOT_S : Inport  Port=10
  RAZ_BY_DIAG : Inport  Port=11  OutDataTypeStr=boolean
      settings: AttributesFormatString=Type : %<OutDataTypeStr>
  NB_PRESENT_DTC_S : Inport  Port=12
  Enable : EnablePort
      settings: AttributesFormatString=State : %<StatesWhenEnabling>
  Constant : Constant  Value=NUMBER_DTC_RECORD_IN_RAM_CST  OutDataTypeStr=uint8  SampleTime=-1
  Constant1 : Constant  Value=NUMBER_DTC_RECORD_IN_E2P_CST  OutDataTypeStr=uint8  SampleTime=-1
  Constant2 : Constant  Value=SNAPSHOT_MAX_LENGHT  OutDataTypeStr=uint8  SampleTime=-1
  Constant3 : Constant  Value=0  OutDataTypeStr=uint32  SampleTime=-1
  Constant4 : Constant  Value=0  OutDataTypeStr=uint8  SampleTime=-1
  Constant5 : Constant  Value=0  OutDataTypeStr=uint32  SampleTime=-1
  Constant6 : Constant  Value=0  OutDataTypeStr=uint8  SampleTime=-1
  Constant7 : Constant  Value=0  OutDataTypeStr=uint8  SampleTime=-1
  EEPROM_chart : Stateflow chart  TreatAsAtomicUnit=on
  Switch{1..5} (5 alike) : Switch  Criteria=u2 ~= 0  RndMeth=Zero  InputSameDT=on
      settings: AttributesFormatString=Criteria=%<Criteria>
  DTC_LIST_OUT_EXT_DATA_S_OUT : Outport
  DTC_LIST_OUT_IDENTITY_DTC_S_OUT : Outport  Port=2
  DTC_LIST_OUT_SNAPSHOT_S_OUT : Outport  Port=3
  DTC_LIST_OUT_OCCUR_CNT_S_OUT : Outport  Port=4
  NB_PRESENT_DTC_S_OUT : Outport  Port=5
  wires:
  TABLE_DTC_ID/1 -> EEPROM_chart/4(DTC_ID)
  SNAPSHOT_TABLE/1 -> EEPROM_chart/8(SNAPSHOT_TABLE)
  TABLE_DTC_SNAPSHOT_NUMBER_CONV/1 -> EEPROM_chart/10(TABLE_DTC_SNAPSHOT_NUMBER_CONV)
  STATUS_TABLE/1 -> EEPROM_chart/9(STATUS_TABLE)
  Switch5/1 -> DTC_LIST_OUT_EXT_DATA_S_OUT/1
  Switch1/1 -> DTC_LIST_OUT_IDENTITY_DTC_S_OUT/1
  Switch2/1 -> DTC_LIST_OUT_SNAPSHOT_S_OUT/1
  Switch3/1 -> DTC_LIST_OUT_OCCUR_CNT_S_OUT/1
  TCONF_CHANGED/1 -> EEPROM_chart/2(TCONF_CHANGED)
  NUMBER_TCONF_UP/1 -> EEPROM_chart/3(NUMBER_TCONF_UP)
  DTC_LIST_OUT_IDENTITY_DTC_S/1 -> EEPROM_chart/5(DTC_LIST_OUT_IDENTITY_DTC_S)
  DTC_LIST_OUT_OCCUR_CNT_S/1 -> EEPROM_chart/6(DTC_LIST_OUT_OCCUR_CNT_S)
  DTC_LIST_OUT_EXT_DATA_S/1 -> EEPROM_chart/11(DTC_LIST_OUT_EXT_DATA_S)
  DTC_LIST_OUT_SNAPSHOT_S/1 -> EEPROM_chart/12(DTC_LIST_OUT_SNAPSHOT_S)
  Constant/1 -> EEPROM_chart/1(NUMBER_DTC_RECORD_IN_RAM)
  Constant1/1 -> EEPROM_chart/7(NUMBER_DTC_RECORD_IN_EEPROM)
  Constant2/1 -> EEPROM_chart/13(SNAPSHOT_MAX_LENGHT)
  Constant5/1 -> Switch5/1
  Constant3/1 -> Switch1/1
  Constant4/1 -> Switch2/1
  Constant6/1 -> Switch3/1
  EEPROM_chart/1(DTC_LIST_OUT_EXT_DATA_S_OUT) -> Switch5/3
  EEPROM_chart/2(DTC_LIST_OUT_IDENTITY_DTC_S_OUT) -> Switch1/3
  EEPROM_chart/3(DTC_LIST_OUT_SNAPSHOT_S_OUT) -> Switch2/3
  EEPROM_chart/4(DTC_LIST_OUT_OCCUR_CNT_S_OUT) -> Switch3/3
  Switch4/1 -> NB_PRESENT_DTC_S_OUT/1
  RAZ_BY_DIAG/1 -> Switch5/2, Switch1/2, Switch2/2, Switch4/2, Switch3/2
  Constant7/1 -> Switch4/1
  EEPROM_chart/5(NB_PRESENT_DTC_S_OUT) -> Switch4/3
  NB_PRESENT_DTC_S/1 -> EEPROM_chart/14(NB_PRESENT_DTC_S)

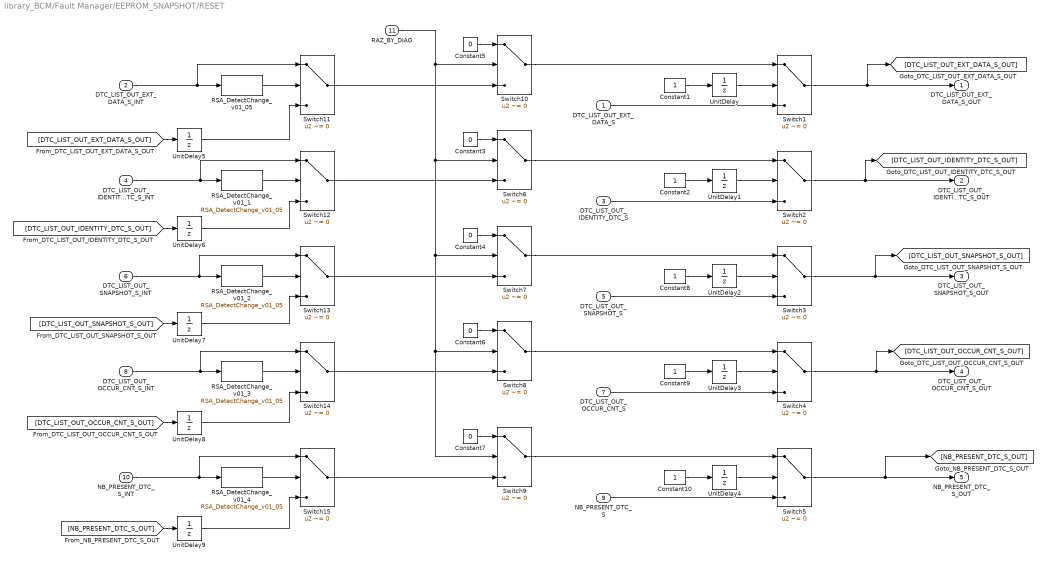
== system library_BCM/Fault Manager/EEPROM_SNAPSHOT/RESET ==
  DTC_LIST_OUT_EXT_DATA_S : Inport  OutDataTypeStr=uint32
      settings: AttributesFormatString=Type : %<OutDataTypeStr>
  DTC_LIST_OUT_EXT_DATA_S_INT : Inport  Port=2  OutDataTypeStr=uint32
      settings: AttributesFormatString=Type : %<OutDataTypeStr>
  DTC_LIST_OUT_IDENTITY_DTC_S : Inport  Port=3  OutDataTypeStr=uint32
      settings: AttributesFormatString=Type : %<OutDataTypeStr>
  DTC_LIST_OUT_IDENTITY_DTC_S_INT : Inport  Port=4  OutDataTypeStr=uint32
      settings: AttributesFormatString=Type : %<OutDataTypeStr>
  DTC_LIST_OUT_SNAPSHOT_S : Inport  Port=5  OutDataTypeStr=uint8
      settings: AttributesFormatString=Type : %<OutDataTypeStr>
  DTC_LIST_OUT_SNAPSHOT_S_INT : Inport  Port=6  OutDataTypeStr=uint8
      settings: AttributesFormatString=Type : %<OutDataTypeStr>
  DTC_LIST_OUT_OCCUR_CNT_S : Inport  Port=7  OutDataTypeStr=uint8
      settings: AttributesFormatString=Type : %<OutDataTypeStr>
  DTC_LIST_OUT_OCCUR_CNT_S_INT : Inport  Port=8  OutDataTypeStr=uint8
      settings: AttributesFormatString=Type : %<OutDataTypeStr>
  NB_PRESENT_DTC_S : Inport  Port=9  OutDataTypeStr=uint8
      settings: AttributesFormatString=Type : %<OutDataTypeStr>
  NB_PRESENT_DTC_S_INT : Inport  Port=10  OutDataTypeStr=uint8
      settings: AttributesFormatString=Type : %<OutDataTypeStr>
  RAZ_BY_DIAG : Inport  Port=11  OutDataTypeStr=boolean
      settings: AttributesFormatString=Type : %<OutDataTypeStr>
  Constant{1..2,8..10} (5 alike) : Constant  OutDataTypeStr=boolean
  Constant3 : Constant  Value=0  OutDataTypeStr=uint32  SampleTime=-1
  Constant4 : Constant  Value=0  OutDataTypeStr=uint8  SampleTime=-1
  Constant5 : Constant  Value=0  OutDataTypeStr=uint32  SampleTime=-1
  Constant6 : Constant  Value=0  OutDataTypeStr=uint8  SampleTime=-1
  Constant7 : Constant  Value=0  OutDataTypeStr=uint8  SampleTime=-1
  RSA_DetectChange_v01_05 : Renault_Library/Complex blocks/Logic & Bit Operations/RSA_DetectChange_v01_05  Tag=[LIB]  chkini=off  vinit=0  tolerance=Absolute Zero  user_tol=0
      settings: AttributesFormatString=|
      | %<MaskType> : Ver : 01.05
      | Compare the Input with Initial Value = %<chkini>
      | Tolerance : %<tolerance>
  RSA_DetectChange_v01_{1..4} (4 alike) : Renault_Library/Complex blocks/Logic & Bit Operations/RSA_DetectChange_v01_05  Tag=[LIB]  chkini=off  vinit=0  tolerance=Absolute Zero  user_tol=0
      settings: AttributesFormatString=|
      | %<MaskType> : Ver : 01.05
      | Compare the Input with Initial Value = %<chkini>
      | Tolerance : %<tolerance>
  Switch{1..15} (15 alike) : Switch  Criteria=u2 ~= 0  RndMeth=Zero  InputSameDT=on
      settings: AttributesFormatString=Criteria=%<Criteria>
  UnitDelay{,1..9} (10 alike) : UnitDelay  SampleTime=-1
      settings: AttributesFormatString=IC = %<X0>
  DTC_LIST_OUT_EXT_DATA_S_OUT : Outport  OutDataTypeStr=uint32
      settings: AttributesFormatString=Type : %<OutDataTypeStr>\nInit :%<InitialOutput>
  DTC_LIST_OUT_IDENTITY_DTC_S_OUT : Outport  Port=2  OutDataTypeStr=uint32
      settings: AttributesFormatString=Type : %<OutDataTypeStr>\nInit :%<InitialOutput>
  DTC_LIST_OUT_SNAPSHOT_S_OUT : Outport  Port=3  OutDataTypeStr=uint8
      settings: AttributesFormatString=Type : %<OutDataTypeStr>\nInit :%<InitialOutput>
  DTC_LIST_OUT_OCCUR_CNT_S_OUT : Outport  Port=4  OutDataTypeStr=uint8
      settings: AttributesFormatString=Type : %<OutDataTypeStr>\nInit :%<InitialOutput>
  NB_PRESENT_DTC_S_OUT : Outport  Port=5  OutDataTypeStr=uint8
      settings: AttributesFormatString=Type : %<OutDataTypeStr>\nInit :%<InitialOutput>
  wires:
  UnitDelay/1 -> Switch1/2
  UnitDelay1/1 -> Switch2/2
  UnitDelay2/1 -> Switch3/2
  UnitDelay3/1 -> Switch4/2
  Switch8/1 -> Switch4/1
  DTC_LIST_OUT_OCCUR_CNT_S/1 -> Switch4/3
  Switch7/1 -> Switch3/1
  DTC_LIST_OUT_SNAPSHOT_S/1 -> Switch3/3
  Switch6/1 -> Switch2/1
  DTC_LIST_OUT_IDENTITY_DTC_S/1 -> Switch2/3
  Switch10/1 -> Switch1/1
  DTC_LIST_OUT_EXT_DATA_S/1 -> Switch1/3
  UnitDelay4/1 -> Switch5/2
  Switch9/1 -> Switch5/1
  NB_PRESENT_DTC_S/1 -> Switch5/3
  Constant5/1 -> Switch10/1
  Constant3/1 -> Switch6/1
  Constant4/1 -> Switch7/1
  Constant6/1 -> Switch8/1
  RAZ_BY_DIAG/1 -> Switch9/2, Switch8/2, Switch7/2, Switch6/2, Switch10/2
  Constant7/1 -> Switch9/1
  Constant1/1 -> UnitDelay/1
  Constant2/1 -> UnitDelay1/1
  Constant8/1 -> UnitDelay2/1
  Constant9/1 -> UnitDelay3/1
  Constant10/1 -> UnitDelay4/1
  Switch11/1 -> Switch10/3
  Switch12/1 -> Switch6/3
  Switch13/1 -> Switch7/3
  Switch14/1 -> Switch8/3
  Switch15/1 -> Switch9/3
  DTC_LIST_OUT_EXT_DATA_S_INT/1 -> Switch11/1, RSA_DetectChange_v01_05/1
  DTC_LIST_OUT_IDENTITY_DTC_S_INT/1 -> Switch12/1, RSA_DetectChange_v01_1/1
  DTC_LIST_OUT_SNAPSHOT_S_INT/1 -> Switch13/1, RSA_DetectChange_v01_2/1
  DTC_LIST_OUT_OCCUR_CNT_S_INT/1 -> Switch14/1, RSA_DetectChange_v01_3/1
  NB_PRESENT_DTC_S_INT/1 -> Switch15/1, RSA_DetectChange_v01_4/1
  RSA_DetectChange_v01_05/1 -> Switch11/2
  RSA_DetectChange_v01_1/1 -> Switch12/2
  RSA_DetectChange_v01_2/1 -> Switch13/2
  RSA_DetectChange_v01_3/1 -> Switch14/2
  RSA_DetectChange_v01_4/1 -> Switch15/2
  UnitDelay5/1 -> Switch11/3
  UnitDelay6/1 -> Switch12/3
  UnitDelay7/1 -> Switch13/3
  UnitDelay8/1 -> Switch14/3
  UnitDelay9/1 -> Switch15/3
  Switch1/1 -> [DTC_LIST_OUT_EXT_DATA_S_OUT], DTC_LIST_OUT_EXT_DATA_S_OUT/1
  Switch2/1 -> [DTC_LIST_OUT_IDENTITY_DTC_S_OUT], DTC_LIST_OUT_IDENTITY_DTC_S_OUT/1
  Switch3/1 -> [DTC_LIST_OUT_SNAPSHOT_S_OUT], DTC_LIST_OUT_SNAPSHOT_S_OUT/1
  Switch4/1 -> [DTC_LIST_OUT_OCCUR_CNT_S_OUT], DTC_LIST_OUT_OCCUR_CNT_S_OUT/1
  Switch5/1 -> [NB_PRESENT_DTC_S_OUT], NB_PRESENT_DTC_S_OUT/1
  [DTC_LIST_OUT_EXT_DATA_S_OUT] -> UnitDelay5/1
  [DTC_LIST_OUT_IDENTITY_DTC_S_OUT] -> UnitDelay6/1
  [DTC_LIST_OUT_SNAPSHOT_S_OUT] -> UnitDelay7/1
  [DTC_LIST_OUT_OCCUR_CNT_S_OUT] -> UnitDelay8/1
  [NB_PRESENT_DTC_S_OUT] -> UnitDelay9/1

== system library_BCM/MIL Full Matlab/Scheduling/Enabled Subsystem ==
  Trigger : TriggerPort
  Function-Call Generator : simulink/Ports & Subsystems/Function-Call Generator  sample_time=-1  numberOfIterations=1
  Out1 : Outport
  wires:
  Function-Call Generator/1 -> Out1/1

== system library_BCM/MIL Full Matlab/Scheduling/Lib_Trigger ==
  Constant1 : Constant  Value=Frequency  OutDataTypeStr=uint32  SampleTime=-1
  Trigger : Subsystem
  Out1 : Outport
      settings: AttributesFormatString=Type : %<OutDataTypeStr>\nInit :%<InitialOutput>
  wires:
  Constant1/1 -> Trigger/1(In1)
  Trigger/1(Out1) -> Out1/1

== system library_BCM/MIL Full Matlab/Scheduling0/Enabled Subsystem ==
  Enable : EnablePort
      settings: AttributesFormatString=State : %<StatesWhenEnabling>
  Function-Call Generator : simulink/Ports & Subsystems/Function-Call Generator  sample_time=-1  numberOfIterations=1
  Out1 : Outport
  wires:
  Function-Call Generator/1 -> Out1/1

== system library_BCM/MIL Full Matlab/Scheduling0/Lib_Trigger ==
  Constant1 : Constant  Value=Frequency  OutDataTypeStr=uint32  SampleTime=-1
  Trigger : Subsystem
  Out1 : Outport
      settings: AttributesFormatString=Type : %<OutDataTypeStr>\nInit :%<InitialOutput>
  wires:
  Trigger/1(Out1) -> Out1/1
  Constant1/1 -> Trigger/1(In1)

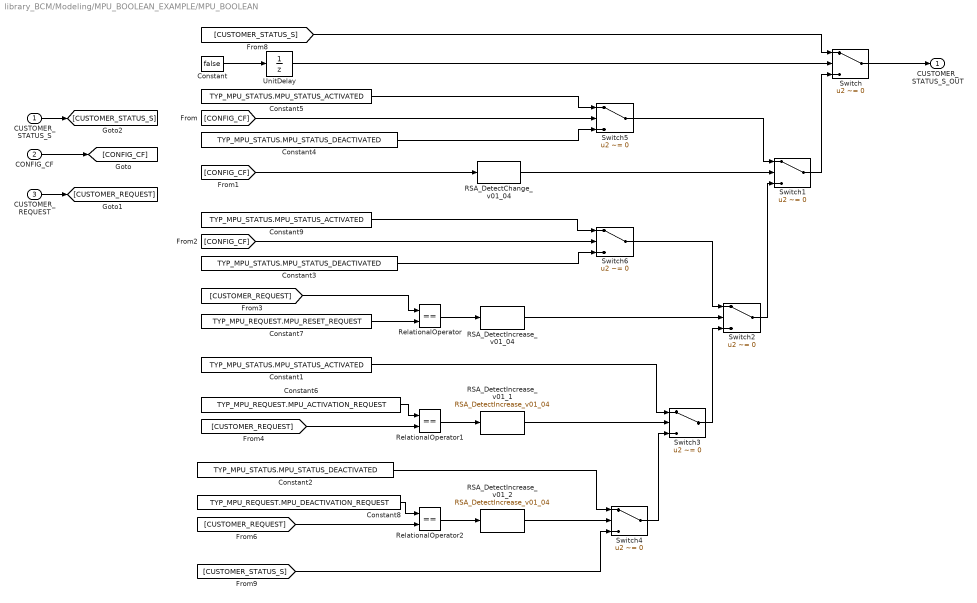
== system library_BCM/Modeling/MPU_BOOLEAN_EXAMPLE/MPU_BOOLEAN ==
  CUSTOMER_STATUS_S : Inport
      settings: AttributesFormatString=Type : %<OutDataTypeStr>
  CONFIG_CF : Inport  Port=2
      settings: AttributesFormatString=Type : %<OutDataTypeStr>
  CUSTOMER_REQUEST : Inport  Port=3
      settings: AttributesFormatString=Type : %<OutDataTypeStr>
  Constant : Constant  Value=false  OutDataTypeStr=boolean  SampleTime=-1
  Constant1 : Constant  Value=TYP_MPU_STATUS.MPU_STATUS_ACTIVATED  OutDataTypeStr=Enum: TYP_MPU_STATUS  SampleTime=-1
  Constant2 : Constant  Value=TYP_MPU_STATUS.MPU_STATUS_DEACTIVATED  OutDataTypeStr=Enum: TYP_MPU_STATUS  SampleTime=-1
  Constant3 : Constant  Value=TYP_MPU_STATUS.MPU_STATUS_DEACTIVATED  OutDataTypeStr=Enum: TYP_MPU_STATUS  SampleTime=-1
  Constant4 : Constant  Value=TYP_MPU_STATUS.MPU_STATUS_DEACTIVATED  OutDataTypeStr=Enum: TYP_MPU_STATUS  SampleTime=-1
  Constant5 : Constant  Value=TYP_MPU_STATUS.MPU_STATUS_ACTIVATED  OutDataTypeStr=Enum: TYP_MPU_STATUS  SampleTime=-1
  Constant6 : Constant  Value=TYP_MPU_REQUEST.MPU_ACTIVATION_REQUEST  OutDataTypeStr=Enum: TYP_MPU_REQUEST  SampleTime=-1
  Constant7 : Constant  Value=TYP_MPU_REQUEST.MPU_RESET_REQUEST  OutDataTypeStr=Enum: TYP_MPU_REQUEST  SampleTime=-1
  Constant8 : Constant  Value=TYP_MPU_REQUEST.MPU_DEACTIVATION_REQUEST  OutDataTypeStr=Enum: TYP_MPU_REQUEST  SampleTime=-1
  Constant9 : Constant  Value=TYP_MPU_STATUS.MPU_STATUS_ACTIVATED  OutDataTypeStr=Enum: TYP_MPU_STATUS  SampleTime=-1
  RSA_DetectChange_v01_04 : Renault_Library/Complex blocks/Logic & Bit Operations/RSA_DetectChange_v01_04  Tag=[LIB]  chkini=off  vinit=0
      settings: AttributesFormatString=%<MaskType> : Ver : 01.04\nCompare the Input with Initial Value = %<chkini>\nInitial Value : = %<vinit>
  RSA_DetectIncrease_v01_04 : Renault_Library/Complex blocks/Logic & Bit Operations/RSA_DetectIncrease_v01_04  Tag=[LIB]  chkini=on  vinit=0
      settings: AttributesFormatString=%<MaskType> : Ver : 01.04\nCompare the Input with Initial Value = %<chkini>\nInitial Value : = %<vinit>
  RSA_DetectIncrease_v01_1 : Renault_Library/Complex blocks/Logic & Bit Operations/RSA_DetectIncrease_v01_04  Tag=[LIB]  chkini=on  vinit=0
      settings: AttributesFormatString=%<MaskType> : Ver : 01.04\nCompare the Input with Initial Value = %<chkini>\nInitial Value : = %<vinit>
  RSA_DetectIncrease_v01_2 : Renault_Library/Complex blocks/Logic & Bit Operations/RSA_DetectIncrease_v01_04  Tag=[LIB]  chkini=on  vinit=0
      settings: AttributesFormatString=%<MaskType> : Ver : 01.04\nCompare the Input with Initial Value = %<chkini>\nInitial Value : = %<vinit>
  RelationalOperator : RelationalOperator  Operator===  OutDataTypeStr=boolean  InputSameDT=on
  RelationalOperator1 : RelationalOperator  Operator===  OutDataTypeStr=boolean  InputSameDT=on
  RelationalOperator2 : RelationalOperator  Operator===  OutDataTypeStr=boolean  InputSameDT=on
  Switch{,1..6} (7 alike) : Switch  Criteria=u2 ~= 0  RndMeth=Zero  InputSameDT=on
      settings: AttributesFormatString=Threshold : %<Threshold>\nSaturation:%<SaturateOnIntegerOverflow>\nCriteria:%<Criteria>
  UnitDelay : UnitDelay  InitialCondition=true  SampleTime=-1
      settings: AttributesFormatString=Initial value : %<X0>
  CUSTOMER_STATUS_S_OUT : Outport
      settings: AttributesFormatString=Init :%<InitialOutput>
  wires:
  Switch6/1 -> Switch2/1
  Constant3/1 -> Switch6/3
  Constant9/1 -> Switch6/1
  [CONFIG_CF] -> Switch6/2
  Switch5/1 -> Switch1/1
  Constant4/1 -> Switch5/3
  Constant5/1 -> Switch5/1
  [CONFIG_CF] -> Switch5/2
  [CUSTOMER_STATUS_S] -> Switch4/3
  [CUSTOMER_STATUS_S] -> Switch/1
  CUSTOMER_STATUS_S/1 -> [CUSTOMER_STATUS_S]
  RSA_DetectIncrease_v01_2/1 -> Switch4/2
  Constant2/1 -> Switch4/1
  Switch4/1 -> Switch3/3
  RelationalOperator2/1 -> RSA_DetectIncrease_v01_2/1
  [CUSTOMER_REQUEST] -> RelationalOperator2/2
  Constant8/1 -> RelationalOperator2/1
  RSA_DetectIncrease_v01_1/1 -> Switch3/2
  Constant1/1 -> Switch3/1
  RelationalOperator1/1 -> RSA_DetectIncrease_v01_1/1
  [CUSTOMER_REQUEST] -> RelationalOperator1/2
  Constant6/1 -> RelationalOperator1/1
  Constant7/1 -> RelationalOperator/2
  Switch3/1 -> Switch2/3
  [CUSTOMER_REQUEST] -> RelationalOperator/1
  CUSTOMER_REQUEST/1 -> [CUSTOMER_REQUEST]
  Switch2/1 -> Switch1/3
  RSA_DetectIncrease_v01_04/1 -> Switch2/2
  RelationalOperator/1 -> RSA_DetectIncrease_v01_04/1
  [CONFIG_CF] -> RSA_DetectChange_v01_04/1
  CONFIG_CF/1 -> [CONFIG_CF]
  RSA_DetectChange_v01_04/1 -> Switch1/2
  Switch1/1 -> Switch/3
  Switch/1 -> CUSTOMER_STATUS_S_OUT/1
  Constant/1 -> UnitDelay/1
  UnitDelay/1 -> Switch/2
